simulink model "cal1"  (R2015a)
settings: Solver=ode45  StartTime=0.0  StopTime=10.0  RelTol=1e-3
undefined symbols (not defined in the file or in its folder): CONST_VAL1
settings Model: Creator=AdminUser  LastModifiedBy=AdminUser

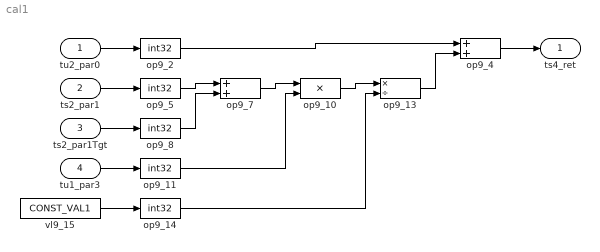
== system cal1 ==
  tu2_par0 : Inport
  ts2_par1 : Inport  Port=2
  ts2_par1Tgt : Inport  Port=3
  tu1_par3 : Inport  Port=4
  op9_10 : Product  Inputs=**
  op9_{2,5,8,11,14} (5 alike) : DataTypeConversion  OutDataTypeStr=int32
  op9_13 : Product  Inputs=*/
  op9_4 : Sum
  op9_7 : Sum
  vl9_15 : Constant  Value=CONST_VAL1
  ts4_ret : Outport
  wires:
  op9_2/1 -> op9_4/1
  op9_13/1 -> op9_4/2
  tu2_par0/1 -> op9_2/1
  op9_10/1 -> op9_13/1
  op9_14/1 -> op9_13/2
  op9_7/1 -> op9_10/1
  op9_11/1 -> op9_10/2
  op9_5/1 -> op9_7/1
  op9_8/1 -> op9_7/2
  ts2_par1/1 -> op9_5/1
  ts2_par1Tgt/1 -> op9_8/1
  tu1_par3/1 -> op9_11/1
  vl9_15/1 -> op9_14/1
  op9_4/1 -> ts4_ret/1
